simulink model "ABLF_SLDO_benchmark"  (R2021b)
settings: Solver=FixedStepAuto  StartTime=0.0  StopTime=100  FixedStep=0.0001  RelTol=1e-3
model workspace (MAT data in the model file):
  SOD_FISP_Test2a_sdosession : sldodialogs.data.SessionData (value not decoded)
values from neighbouring files (symbols this model uses):
  a = 2    [ABLF_SLDO_benchmark_Start.m]    (also in ABLF_SOC_benchmark_Start.m)
  f1 = 0    [ABLF_SLDO_benchmark_Start.m]    (also in ABLF_SOC_benchmark_Start.m)
  g1 = 1    [ABLF_SLDO_benchmark_Start.m]    (also in ABLF_SOC_benchmark_Start.m)
  g2 = Kt/J    (= 0.530555555556)    [ABLF_SLDO_benchmark_Start.m]    (also in ABLF_SOC_benchmark_Start.m)
  g3 = 1/L    (= 333.333333333)    [ABLF_SLDO_benchmark_Start.m]    (also in ABLF_SOC_benchmark_Start.m)
  J = 1.8*10^(-2)    (= 0.018)    [ABLF_SLDO_benchmark_Start.m]    (also in ABLF_SOC_benchmark_Start.m)
  k = 2    [ABLF_SLDO_benchmark_Start.m]    (also in ABLF_SOC_benchmark_Start.m)
  k1 = 6.2718    [ABLF_SLDO_benchmark_Start.m]    (also in ABLF_SOC_benchmark_Start.m = 10)
  k2 = 2.3993e+03    (= 2399.3)    [ABLF_SLDO_benchmark_Start.m]    (also in ABLF_SOC_benchmark_Start.m = 1)
  k3 = 31.9167    [ABLF_SLDO_benchmark_Start.m]    (also in ABLF_SOC_benchmark_Start.m = 10)
  ka1 = kcl1 - (-amp)    (= -0.429203673205)    [ABLF_SLDO_benchmark_Start.m]    (also in ABLF_SOC_benchmark_Start.m = kcl1 - (-amp))
  kb1 = kcl2 - (amp)    (= 0.429203673205)    [ABLF_SLDO_benchmark_Start.m]    (also in ABLF_SOC_benchmark_Start.m = kcl2 - (amp))
  Ke = 9.55*10^(-3)    (= 0.00955)    [ABLF_SLDO_benchmark_Start.m]    (also in ABLF_SOC_benchmark_Start.m)
  Kt = 9.55*10^(-3)    (= 0.00955)    [ABLF_SLDO_benchmark_Start.m]    (also in ABLF_SOC_benchmark_Start.m)
  L = 0.003    [ABLF_SLDO_benchmark_Start.m]    (also in ABLF_SOC_benchmark_Start.m = 1)
  mu1 = 1.8    [ABLF_SLDO_benchmark_Start.m]    (also in ABLF_SOC_benchmark_Start.m)
  R = 0.21    [ABLF_SLDO_benchmark_Start.m]    (also in ABLF_SOC_benchmark_Start.m)
  t2 = 0.012    [ABLF_SLDO_benchmark_Start.m]    (also in ABLF_SOC_benchmark_Start.m = 0.0005)
  t3 = 0.012    [ABLF_SLDO_benchmark_Start.m]    (also in ABLF_SOC_benchmark_Start.m = 0.01)
settings Model: Creator=mcald  LastModifiedBy=mcald
settings DataIOCC: ReturnWorkspaceOutputs=off  ReturnWorkspaceOutputsName=SDOSimTest_Log

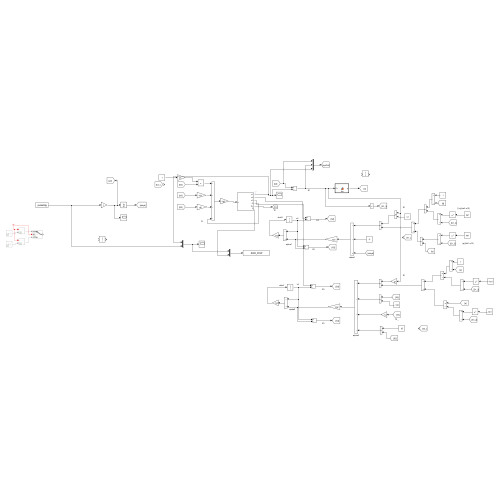
[thumbnail: Simulink's stored preview of the top-level diagram]
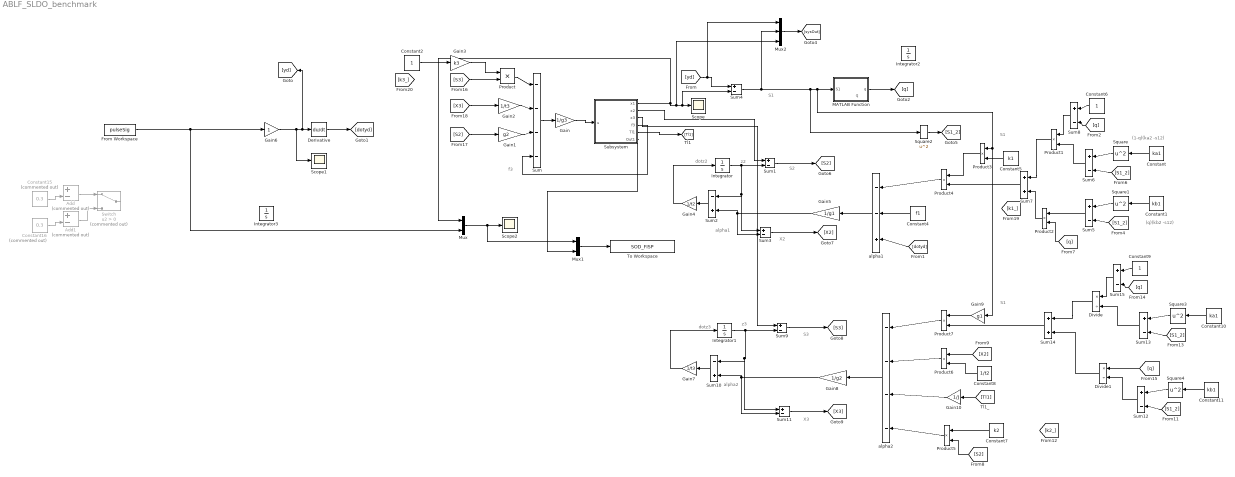
== system ABLF_SLDO_benchmark ==
  note: dotz3
  note: X3
  note: alpha1
  note: alpha2
  note: S1
  note: f3
  note: S3
  note: (1-q)(ka2 -s12)
  note: z2
  note: z3
  note: q
  note: S1
  note: X2
  note: S1
  note: dotz2
  note: S2
  note: (q)(kb2 -s12)
  Add : Sum  Commented=on  Inputs=+-
  Add1 : Sum  Commented=on  Inputs=+-
  Constant : Constant  Value=ka1
  Constant1 : Constant  Value=kb1
  Constant10 : Constant  Value=ka1
  Constant11 : Constant  Value=kb1
  Constant15 : Constant  Commented=on  Value=0.3
  Constant16 : Constant  Commented=on  Value=0.3
  Constant2 : Constant
  Constant4 : Constant  Value=f1
  Constant5 : Constant  Value=k1
  Constant6 : Constant
  Constant7 : Constant  Value=k2
  Constant8 : Constant  Value=1/t2
  Constant9 : Constant
  Derivative : Derivative
  Divide : Product  Inputs=*/
  Divide1 : Product  Inputs=*/
  From Workspace : FromWorkspace  VariableName=pulseSig
  Gain : Gain  Gain=1/g3
  Gain1 : Gain  Gain=g2
  Gain10 : Gain  Gain=1/J
  Gain2 : Gain  Gain=1/t3
  Gain3 : Gain  Gain=k3
  Gain4 : Gain  Gain=1/t2
  Gain5 : Gain  Gain=1/g1
  Gain6 : Gain
  Gain7 : Gain  Gain=1/t3
  Gain8 : Gain  Gain=1/g2
  Gain9 : Gain  Gain=g1
  Integrator : Integrator  InitialCondition=-5.0078
  Integrator1 : Integrator  InitialCondition=-2094.2231
  Integrator2 : Integrator
  Integrator3 : Integrator  InitialCondition=0.1
  MATLAB Function : MATLAB Function  TreatAsAtomicUnit=on
  Mux : Mux  Inputs=2
  Mux1 : Mux  Inputs=2
  Mux2 : Mux  Inputs=3
  Product{,1..7} (8 alike) : Product
  Scope : Scope
  Scope1 : Scope
  Scope2 : Scope
  Square{,1..4} (5 alike) : Math  Operator=square  SaturateOnIntegerOverflow=on
  Subsystem : Subsystem
  Sum : Sum  Inputs=-|-|-|-
  Sum{1,3..6,8..9,11..13,15} (11 alike) : Sum  Inputs=+|-
  Sum10 : Sum  Inputs=-|+
  Sum14 : Sum  Inputs=+|+
  Sum2 : Sum  Inputs=-|+
  Sum7 : Sum  Inputs=+|+
  Switch : Switch  Commented=on  Criteria=u2 > Threshold
  To Workspace : ToWorkspace  VariableName=SOD_FISP  SaveFormat=Timeseries  SampleTime=-1
  alpha1 : Sum  Inputs=-|-|+
  alpha2 : Sum  Inputs=-|-|-|-
  wires:
  Sum3/1 -> [X2]
  Gain4/1 -> Integrator/1
  Constant/1 -> Square/1
  Sum4/1 -> Square2/1, Gain9/1, Product3/1, MATLAB Function/1(S1), Mux2/2
  Product/1 -> Sum/1
  Constant2/1 -> Gain3/1
  Subsystem/5(Tl1) -> [Tl1]
  [S1_2] -> Sum13/2
  Divide/1 -> Sum14/1
  Constant16/1 -> Add1/2
  Subsystem/1(x1) -> Mux2/3, Sum4/2, Scope/1, Mux/1
  Gain10/1 -> alpha2/3
  Gain9/1 -> Product7/1
  Gain2/1 -> Sum/2
  Sum7/1 -> Product4/2
  Constant1/1 -> Square1/1
  Square/1 -> Sum6/1
  MATLAB Function/1(q) -> [q]
  [S3] -> Product/2
  Constant10/1 -> Square3/1
  Square4/1 -> Sum12/1
  [S2] -> Gain1/1
  Integrator/1 -> Sum3/1, Sum2/1, Sum1/2
  Gain1/1 -> Sum/3
  Sum9/1 -> [S3]
  [X3] -> Gain2/1
  [q] -> Sum8/2
  Constant7/1 -> Product5/1
  Mux/1 -> Mux1/1, Scope2/1
  Constant11/1 -> Square4/1
  Product2/1 -> Sum7/2
  Subsystem/3(x3) -> Sum9/1
  Divide1/1 -> Sum14/2
  [dotyd] -> alpha1/3
  Sum15/1 -> Divide/1
  Gain6/1 -> Derivative/1, [yd], Scope1/1
  Product6/1 -> alpha2/2
  Sum12/1 -> Divide1/2
  Sum14/1 -> Product7/2
  [q] -> Sum15/2
  Constant5/1 -> Product3/2
  Constant6/1 -> Sum8/1
  [q] -> Divide1/1
  [S1_2] -> Sum6/2
  Gain/1 -> Subsystem/1(u)
  Product5/1 -> alpha2/4
  Sum5/1 -> Product2/1
  Square2/1 -> [S1_2]
  Sum13/1 -> Divide/2
  Gain5/1 -> Sum2/2, Sum3/2
  Sum11/1 -> [X3]
  Gain3/1 -> Product/1
  Square3/1 -> Sum13/1
  Add/1 -> Switch/1
  Mux2/1 -> [sysOut]
  Product1/1 -> Sum7/1
  Derivative/1 -> [dotyd]
  Product7/1 -> alpha2/1
  Constant15/1 -> Add/2
  Gain8/1 -> Sum10/2, Sum11/2
  Constant8/1 -> Product6/2
  alpha2/1 -> Gain8/1
  [S1_2] -> Sum12/2
  Subsystem/4(f3) -> Sum/4
  Product3/1 -> Product4/1
  Sum8/1 -> Product1/1
  Sum/1 -> Gain/1
  Subsystem/2(x2) -> Sum1/1
  Constant9/1 -> Sum15/1
  Add1/1 -> Switch/3
  [Tl1] -> Gain10/1
  [S1_2] -> Sum5/2
  Sum2/1 -> Gain4/1
  [X2] -> Product6/1
  Gain7/1 -> Integrator1/1
  From Workspace/1 -> Mux/2, Gain6/1
  Sum1/1 -> [S2]
  Product4/1 -> alpha1/1
  Sum6/1 -> Product1/2
  Integrator1/1 -> Sum11/1, Sum10/1, Sum9/2
  [yd] -> Mux2/1, Sum4/1
  Sum10/1 -> Gain7/1
  ? -> Switch/2
  ? -> Add1/1, Add/1
  [S2] -> Product5/2
  Square1/1 -> Sum5/1
  Constant4/1 -> alpha1/2
  [q] -> Product2/2
  alpha1/1 -> Gain5/1
  Mux1/1 -> To Workspace/1
  Subsystem/6(Out1) -> Mux1/2

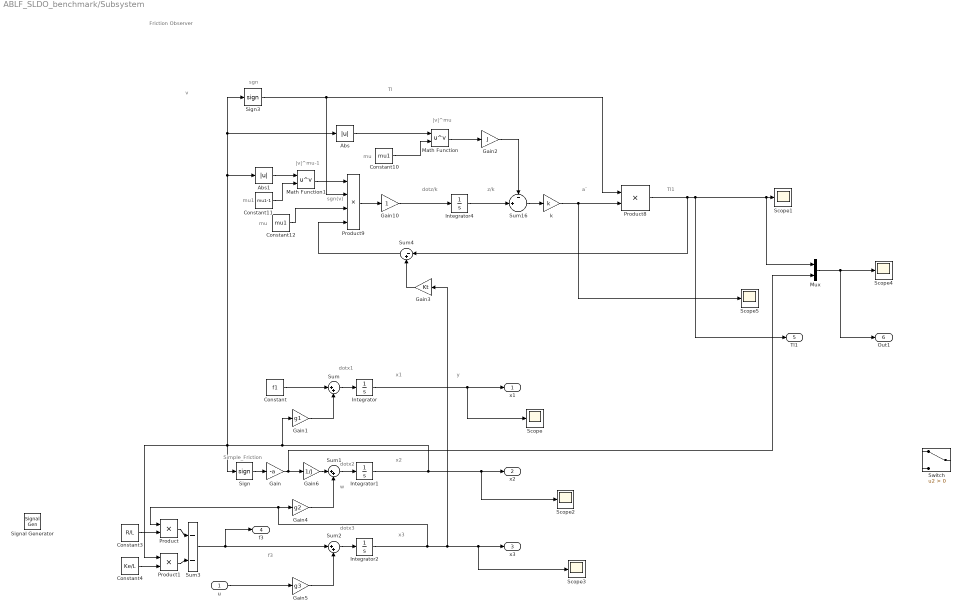
== system ABLF_SLDO_benchmark/Subsystem ==
  note: Simple_Friction
  note: w
  note: Tl
  note: f3
  note: y
  note: x1
  note: dotx1
  note: dotx2
  note: x2
  note: dotx3
  note: x3
  note: mu1
  note: dotz/k
  note: v
  note: mu
  note: a`
  note: z/k
  note: sgn
  note: Friction Observer
  note: mu
  note: |v|^mu-1
  note: sgn(v)
  note: |v|^mu
  note: Tl1
  u : Inport
  Abs : Abs
  Abs1 : Abs
  Constant : Constant  Value=f1
  Constant10 : Constant  Value=mu1
  Constant11 : Constant  Value=mu1-1
  Constant12 : Constant  Value=mu1
  Constant3 : Constant  Value=R/L
  Constant4 : Constant  Value=Ke/L
  Gain : Gain  Gain=-a
  Gain1 : Gain  Gain=g1
  Gain10 : Gain
  Gain2 : Gain  Gain=J
  Gain3 : Gain  Gain=Kt
  Gain4 : Gain  Gain=g2
  Gain5 : Gain  Gain=g3
  Gain6 : Gain  Gain=1/J
  Integrator : Integrator  InitialCondition=0.1
  Integrator1 : Integrator  InitialCondition=0.1
  Integrator2 : Integrator  InitialCondition=0.1
  Integrator4 : Integrator  InitialCondition=1
  Math Function : Math  Operator=pow  SaturateOnIntegerOverflow=on
  Math Function1 : Math  Operator=pow  SaturateOnIntegerOverflow=on
  Mux : Mux  Inputs=2
  Product : Product
  Product1 : Product
  Product8 : Product
  Product9 : Product  Inputs=4
  Scope{,1..5} (6 alike) : Scope
  Sign : Signum
  Sign3 : Signum
  Signal Generator : SignalGenerator  WaveForm=square  Amplitude=pi/2  Frequency=0.1  Units=rad/sec
  Sum : Sum  Inputs=|++
  Sum1 : Sum  Inputs=|++
  Sum16 : Sum  Inputs=-|+||
  Sum2 : Sum  Inputs=|++
  Sum3 : Sum  Inputs=-|-
  Sum4 : Sum  Inputs=|-+
  Switch : Switch  Criteria=u2 > Threshold
  k : Gain  Gain=k
  x1 : Outport
  x2 : Outport  Port=2
  x3 : Outport  Port=3
  f3 : Outport  Port=4
  Tl1 : Outport  Port=5
  Out1 : Outport  Port=6
  wires:
  Gain1/1 -> Sum/2
  Gain5/1 -> Sum2/2
  Integrator/1 -> Scope/1, x1/1
  Sum2/1 -> Integrator2/1
  Sum3/1 -> f3/1, Sum2/1
  Constant/1 -> Sum/1
  Sum1/1 -> Integrator1/1
  Integrator2/1 -> Gain3/1, Scope3/1, x3/1, Product/1, Gain4/1
  Sum/1 -> Integrator/1
  Constant3/1 -> Product/2
  Product/1 -> Sum3/1
  Product1/1 -> Sum3/2
  Constant4/1 -> Product1/2
  Integrator4/1 -> Sum16/2
  Abs1/1 -> Math Function1/1
  Math Function1/1 -> Product9/1
  Abs/1 -> Math Function/1
  Product9/1 -> Gain10/1
  Sum16/1 -> k/1
  Gain10/1 -> Integrator4/1
  Sign3/1 -> Product9/2, Product8/1
  Constant12/1 -> Product9/3
  Constant10/1 -> Math Function/2
  k/1 -> Scope5/1, Product8/2
  Constant11/1 -> Math Function1/2
  Sign/1 -> Gain/1
  Gain4/1 -> Sum1/2
  u/1 -> Gain5/1
  Math Function/1 -> Gain2/1
  Gain2/1 -> Sum16/1
  Mux/1 -> Out1/1, Scope4/1
  Product8/1 -> Sum4/1, Tl1/1, Mux/1, Scope1/1
  Gain/1 -> Mux/2, Gain6/1
  Integrator1/1 -> Gain1/1, Abs1/1, Abs/1, Sign3/1, Sign/1, Product1/1, Scope2/1, x2/1
  Gain3/1 -> Sum4/2
  Sum4/1 -> Product9/4
  Gain6/1 -> Sum1/1

== matlab function ABLF_SLDO_benchmark/MATLAB Function ==
  data: S1 input; q output
function q = fcn(S1)
if S1 <= 0
    q = 0;
else  
    q = 1;
end
